simulink model "jav1pitch"  (R2025b)
settings: Solver=VariableStepAuto  StartTime=0.0  StopTime=41  RelTol=1e-3
undefined symbols (not defined in the file): Cd, delta_pitch_saturation, diameter, g, I_treghet, K_finne, Ki_altitude, Kp_altitude, L_aksial, m, rho, T, theta0, theta_dot, theta_ref_saturation, v_x0, v_z0, x0, z0, z_ref
libraries: slpidlib x2
settings Model: Creator=Tobias Stenberg  LastModifiedBy=kristiangjestad

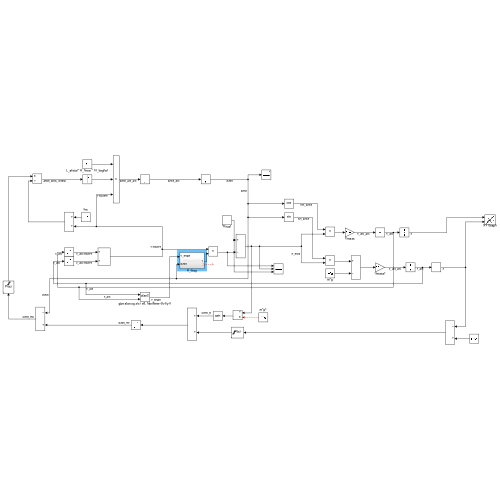
[thumbnail: Simulink's stored preview of the top-level diagram]
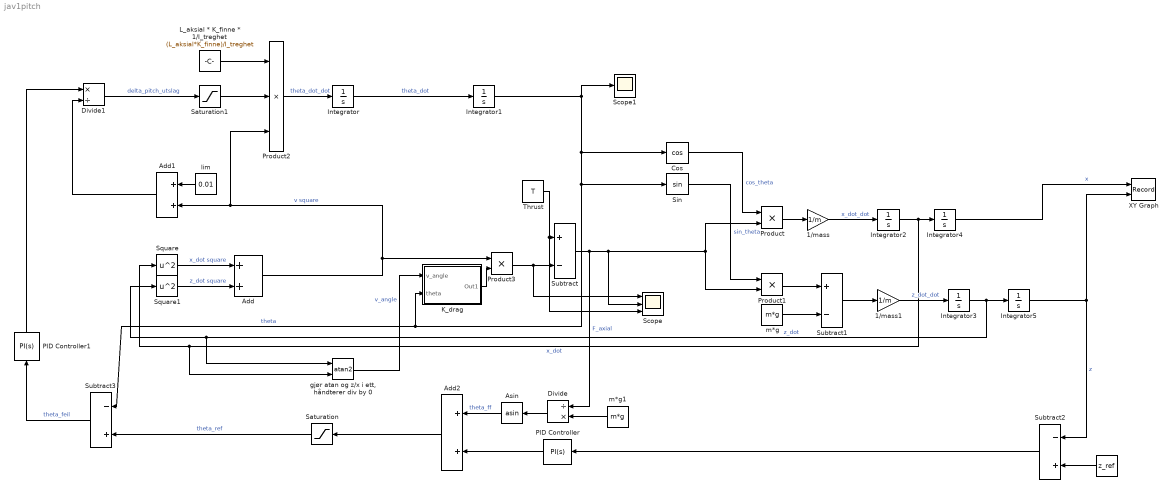
== system jav1pitch ==
  " " : Constant  Value=z_ref
  1/mass : Gain  Gain=1/m
  1/mass1 : Gain  Gain=1/m
  Add : Sum
  Add1 : Sum
  Add2 : Sum
  Asin : Trigonometry  Operator=asin
  Cos : Trigonometry  Operator=cos
  Divide : Product  Inputs=/*
  Divide1 : Product  Inputs=*/
  Integrator : Integrator  InitialCondition=theta_dot
  Integrator1 : Integrator  InitialCondition=theta0
  Integrator2 : Integrator  InitialCondition=v_x0
  Integrator3 : Integrator  InitialCondition=v_z0
  Integrator4 : Integrator  InitialCondition=x0
  Integrator5 : Integrator  InitialCondition=z0
  K_drag : Subsystem
  L_aksial * K_finne * 1/I_treghet : Constant  Value=(L_aksial*K_finne)/I_treghet
  PID Controller : slpidlib/PID Controller  Controller=PI  Form=Parallel  TimeDomain=Continuous-time  UseExternalTs=off  SampleTime=-1  IntegratorMethod=Forward Euler  FilterMethod=Forward Euler  ControllerParametersSource=internal  P=Kp_altitude  I=Ki_altitude  UseKiTs=off  D=0  UseExternalDerivativeSource=off  N=100  UseFilter=on  TunerSelectOption=Transfer Function Based (PID Tuner App)  InitialConditionSource=internal  InitialConditionForIntegrator=0  InitialConditionForFilter=0  DifferentiatorICPrevScaledInput=0  ExternalReset=none  TrackingMode=off  Kt=1  LimitOutput=on  SatLimitsSource=internal  UpperSaturationLimit=0.4  LowerSaturationLimit=-0.4  LinearizeAsGain=on  AntiWindupMode=clamping  Kb=1  LimitIntegrator=off  UpperIntegratorSaturationLimit=inf  LowerIntegratorSaturationLimit=-inf  POutMin=[]  POutMax=[]  IOutMin=[]  IOutMax=[]  DOutMin=[]  DOutMax=[]  NOutMin=[]  NOutMax=[]  SumOutMin=[]  SumOutMax=[]  SaturationOutMin=[]  SaturationOutMax=[]  PParamMin=[]  PParamMax=[]  IParamMin=[]  IParamMax=[]  DParamMin=[]  DParamMax=[]  NParamMin=[]  NParamMax=[]  KbParamMin=[]  KbParamMax=[]  KtParamMin=[]  KtParamMax=[]  KbOutMin=[]  KbOutMax=[]  KtOutMin=[]  KtOutMax=[]  IntegratorOutMin=[]  IntegratorOutMax=[]  FilterOutMin=[]  FilterOutMax=[]  SumI1OutMin=[]  SumI1OutMax=[]  SumI2OutMin=[]  SumI2OutMax=[]  SumI3OutMin=[]  SumI3OutMax=[]  SumI4OutMin=[]  SumI4OutMax=[]  SumDOutMin=[]  SumDOutMax=[]  DifferentiatorOutMin=[]  DifferentiatorOutMax=[]  FilterDiffOutCoefMin=[]  FilterDiffOutCoefMax=[]  ReciprocalOutMin=[]  ReciprocalOutMax=[]  SumDenOutMin=[]  SumDenOutMax=[]  SumNumOutMin=[]  SumNumOutMax=[]  DivideOutMin=[]  DivideOutMax=[]  UdiffTsProdOutMin=[]  UdiffTsProdOutMax=[]  NTsProdOutMin=[]  NTsProdOutMax=[]  UintegralTsProdOutMin=[]  UintegralTsProdOutMax=[]  UngainTsProdOutMin=[]  UngainTsProdOutMax=[]  ClampingZeroOutDataTypeStr=Inherit: Inherit via back propagation  ClampingZeroOutMin=[]  ClampingZeroOutMax=[]  FilterDenConstantOutDataTypeStr=Inherit: Inherit via back propagation  FilterDenConstantOutMin=[]  FilterDenConstantOutMax=[]  PCopyOutDataTypeStr=Inherit: Inherit via back propagation  PCopyOutMin=[]  PCopyOutMax=[]  NCopyOutDataTypeStr=Inherit: Inherit via back propagation  NCopyOutMin=[]  NCopyOutMax=[]  IntegratorContinuousStateAttributes=''  IntegratorStateMustResolveToSignalObject=off  IntegratorRTWStateStorageClass=Auto  FilterContinuousStateAttributes=''  FilterStateMustResolveToSignalObject=off  FilterRTWStateStorageClass=Auto  ParallelPVariant=InternalParameters  IdealPVariant=Disabled  IVariant=InternalParameters  DVariant=Disabled  IntegratorVariant=Continuous  SatVariant=Enabled  AWVariant=ContClampingParallel  PCopyVariant=Disabled  TRVariant=Disabled  FdbkBlocksVariant=Forward  IdealPFdbkVariant=Disabled  SatFdbkVariant=Disabled  DerivativeFilterVariant=Disabled  NVariant=Disabled  NCopyVariant=Disabled_SignalSpec  FilterICVariant=Disabled  IntegratorICVariant=InternalICs  ExternalResetVariant=Disabled  TRSumVariant=Passthrough  SumFdbkVariant=Disabled  SumVariant=Sum_PI  TsampFilterVariant=InternalTs  TsampNgainVariant=Passthrough  TsampIntegralVariant=Disabled_SignalSpec  ExternalSaturationOutDataTypeStr=Inherit: Same as second input  DerivativeSourceVariant=Disabled  PreIntVariant=InternalPreInt
  PID Controller1 : slpidlib/PID Controller  Controller=PI  Form=Parallel  TimeDomain=Continuous-time  UseExternalTs=off  SampleTime=-1  IntegratorMethod=Forward Euler  FilterMethod=Forward Euler  ControllerParametersSource=internal  P=Kp_altitude  I=Ki_altitude  UseKiTs=off  D=0  UseExternalDerivativeSource=off  N=100  UseFilter=on  TunerSelectOption=Transfer Function Based (PID Tuner App)  InitialConditionSource=internal  InitialConditionForIntegrator=0  InitialConditionForFilter=0  DifferentiatorICPrevScaledInput=0  ExternalReset=none  TrackingMode=off  Kt=1  LimitOutput=on  SatLimitsSource=internal  UpperSaturationLimit=0.4  LowerSaturationLimit=-0.4  LinearizeAsGain=on  AntiWindupMode=clamping  Kb=1  LimitIntegrator=off  UpperIntegratorSaturationLimit=inf  LowerIntegratorSaturationLimit=-inf  POutMin=[]  POutMax=[]  IOutMin=[]  IOutMax=[]  DOutMin=[]  DOutMax=[]  NOutMin=[]  NOutMax=[]  SumOutMin=[]  SumOutMax=[]  SaturationOutMin=[]  SaturationOutMax=[]  PParamMin=[]  PParamMax=[]  IParamMin=[]  IParamMax=[]  DParamMin=[]  DParamMax=[]  NParamMin=[]  NParamMax=[]  KbParamMin=[]  KbParamMax=[]  KtParamMin=[]  KtParamMax=[]  KbOutMin=[]  KbOutMax=[]  KtOutMin=[]  KtOutMax=[]  IntegratorOutMin=[]  IntegratorOutMax=[]  FilterOutMin=[]  FilterOutMax=[]  SumI1OutMin=[]  SumI1OutMax=[]  SumI2OutMin=[]  SumI2OutMax=[]  SumI3OutMin=[]  SumI3OutMax=[]  SumI4OutMin=[]  SumI4OutMax=[]  SumDOutMin=[]  SumDOutMax=[]  DifferentiatorOutMin=[]  DifferentiatorOutMax=[]  FilterDiffOutCoefMin=[]  FilterDiffOutCoefMax=[]  ReciprocalOutMin=[]  ReciprocalOutMax=[]  SumDenOutMin=[]  SumDenOutMax=[]  SumNumOutMin=[]  SumNumOutMax=[]  DivideOutMin=[]  DivideOutMax=[]  UdiffTsProdOutMin=[]  UdiffTsProdOutMax=[]  NTsProdOutMin=[]  NTsProdOutMax=[]  UintegralTsProdOutMin=[]  UintegralTsProdOutMax=[]  UngainTsProdOutMin=[]  UngainTsProdOutMax=[]  ClampingZeroOutDataTypeStr=Inherit: Inherit via back propagation  ClampingZeroOutMin=[]  ClampingZeroOutMax=[]  FilterDenConstantOutDataTypeStr=Inherit: Inherit via back propagation  FilterDenConstantOutMin=[]  FilterDenConstantOutMax=[]  PCopyOutDataTypeStr=Inherit: Inherit via back propagation  PCopyOutMin=[]  PCopyOutMax=[]  NCopyOutDataTypeStr=Inherit: Inherit via back propagation  NCopyOutMin=[]  NCopyOutMax=[]  IntegratorContinuousStateAttributes=''  IntegratorStateMustResolveToSignalObject=off  IntegratorRTWStateStorageClass=Auto  FilterContinuousStateAttributes=''  FilterStateMustResolveToSignalObject=off  FilterRTWStateStorageClass=Auto  ParallelPVariant=InternalParameters  IdealPVariant=Disabled  IVariant=InternalParameters  DVariant=Disabled  IntegratorVariant=Continuous  SatVariant=Enabled  AWVariant=ContClampingParallel  PCopyVariant=Disabled  TRVariant=Disabled  FdbkBlocksVariant=Forward  IdealPFdbkVariant=Disabled  SatFdbkVariant=Disabled  DerivativeFilterVariant=Disabled  NVariant=Disabled  NCopyVariant=Disabled_SignalSpec  FilterICVariant=Disabled  IntegratorICVariant=InternalICs  ExternalResetVariant=Disabled  TRSumVariant=Passthrough  SumFdbkVariant=Disabled  SumVariant=Sum_PI  TsampFilterVariant=InternalTs  TsampNgainVariant=Passthrough  TsampIntegralVariant=Disabled_SignalSpec  ExternalSaturationOutDataTypeStr=Inherit: Same as second input  DerivativeSourceVariant=Disabled  PreIntVariant=InternalPreInt
  Product : Product
  Product1 : Product
  Product2 : Product  Inputs=3
  Product3 : Product
  Saturation : Saturate  UpperLimit=theta_ref_saturation  LowerLimit=-theta_ref_saturation
  Saturation1 : Saturate  UpperLimit=delta_pitch_saturation  LowerLimit=-delta_pitch_saturation
  Scope : Scope  NumInputPorts=3
      settings: ActiveDisplayYMinimum=-272.68668201615378  ActiveDisplayYMaximum=1772.6866820161538
  Scope1 : Scope
      settings: ActiveDisplayYMinimum=-0.77176160217650369  ActiveDisplayYMaximum=0.51854075550484957
  Sin : Trigonometry
  Square : Math  Operator=square
  Square1 : Math  Operator=square
  Subtract : Sum  Inputs=+-
  Subtract1 : Sum  Inputs=+-
  Subtract2 : Sum  Inputs=-+
  Subtract3 : Sum  Inputs=-+
  Thrust : Constant  Value=T
  XY Graph : Record  NumPorts=2.0  FileSettingsInternal="{\"entries\":[{\"content\":{\"excelSettings\":{\"content\":{},\"type\":\"Streamout.ExcelSettings\"},\"parquetSettings\":{\"content\":{},\"type\":\"Streamout.ParquetSettings\"}},\"type\":\"Streamout.FileSettingStorage\",\"uuid\":\"\"}],\"packageUris\":[\"http:\\/\\/schema.mathworks.com\\/mf0\\/streamout_blocks\\/R2020a\"],\"version\":\"1.0\"}"  FrameSettings=[0, 0]  Layout=[1 1]  SignalsInternal="{\"entries\":[{\"content\":{\"signals\":[{\"content\":{\"blockPath\":[],\"dimensions\":[1],\"domain\":\"\",\"lineColor\":\"#a2142f\",\"port\":1,\"sid\":[\"\"],\"signalID\":1,\"signalName\":\"x\"},\"type\":\"RecordBlkView.Signal\",\"uuid\":\"\"},{\"content\":{\"blockPath\":[],\"dimensions\":[1],\"domain\":\"\",\"lineColor\":\"#139fff\",\"plots\":[ 1 ],\"port\":2,\"sid\":[\"\"],\"signalID\":2,\"signalName\":\"z\"},\"type\":\"RecordBlkView.Signal\",\"uuid\":\"\"}]},\"type\":\"RecordBlkView.InputSignals\",\"uuid\":\"\"}],\"packageUris\":[\"http:\\/\\/schema.mathworks.com\\/mf0\\/streamout_blocks\\/R2020a\"],\"version\":\"1.0\"}"  CompatibilityTag=XY
  "gjør atan og z/x i ett, håndterer div by 0" : Trigonometry  Operator=atan2
  lim : Constant  Value=0.01
  m*g : Constant  Value=m*g
  m*g1 : Constant  Value=m*g
  wires:
  Integrator/1 -> Integrator1/1  "theta_dot"
  Product2/1 -> Integrator/1  "theta_dot_dot"
  Integrator1/1 -> Sin/1, K_drag/2(theta), Subtract3/1, Cos/1, Scope1/1  "theta"
  Square/1 -> Add/1  "x_dot square"
  Square1/1 -> Add/2  "z_dot square"
  Add/1 -> Product2/3, Add1/2, Product3/1  "v square"
  Product3/1 -> Subtract/2, Scope/1
  Thrust/1 -> Scope/3, Subtract/1
  Subtract/1 -> Divide/1, Scope/2, Product1/2, Product/2  "F_axial"
  Cos/1 -> Product/1  "cos_theta"
  Sin/1 -> Product1/1  "sin_theta"
  Product1/1 -> Subtract1/1
  m*g/1 -> Subtract1/2
  Subtract1/1 -> 1/mass1/1
  1/mass1/1 -> Integrator3/1  "z_dot_dot"
  Product/1 -> 1/mass/1
  1/mass/1 -> Integrator2/1  "x_dot_dot"
  Integrator2/1 -> "gjør atan og z/x i ett, håndterer div by 0"/2, Square/1, Integrator4/1  "x_dot"
  Integrator3/1 -> "gjør atan og z/x i ett, håndterer div by 0"/1, Square1/1, Integrator5/1  "z_dot"
  Integrator4/1 -> XY Graph/1  "x"
  Integrator5/1 -> XY Graph/2, Subtract2/1  "z"
  L_aksial * K_finne * 1/I_treghet/1 -> Product2/1
  Divide1/1 -> Saturation1/1  "delta_pitch_utslag"
  m*g1/1 -> Divide/2
  Divide/1 -> Asin/1
  Asin/1 -> Add2/1  "theta_ff"
  lim/1 -> Add1/1
  Add1/1 -> Divide1/2
  Saturation/1 -> Subtract3/2  "theta_ref"
  Add2/1 -> Saturation/1
  " "/1 -> Subtract2/2
  PID Controller/1 -> Add2/2
  Subtract2/1 -> PID Controller/1
  Subtract3/1 -> PID Controller1/1  "theta_feil"
  Saturation1/1 -> Product2/2
  PID Controller1/1 -> Divide1/1
  "gjør atan og z/x i ett, håndterer div by 0"/1 -> K_drag/1(v_angle)  "v_angle"
  K_drag/1(Out1) -> Product3/2
  ? -> ?

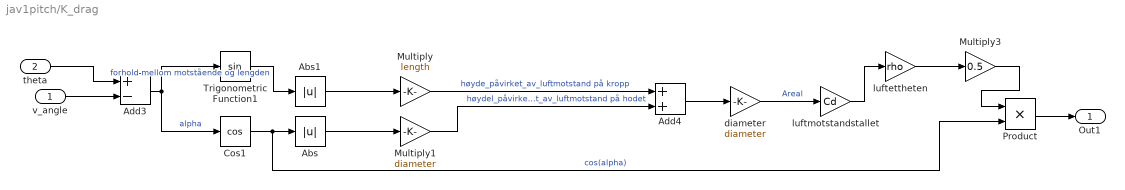
== system jav1pitch/K_drag ==
  v_angle : Inport
  theta : Inport  Port=2
  Abs : Abs  SaturateOnIntegerOverflow=off
  Abs1 : Abs  SaturateOnIntegerOverflow=off
  Add3 : Sum  Inputs=+-
  Add4 : Sum
  Cos1 : Trigonometry  Operator=cos
  Multiply : Gain  Gain=length
  Multiply1 : Gain  Gain=diameter
  Multiply3 : Gain  Gain=0.5
  Product : Product
  Trigonometric Function1 : Trigonometry
  diameter : Gain  Gain=diameter
  luftettheten : Gain  Gain=rho
  luftmotstandstallet : Gain  Gain=Cd
  Out1 : Outport
  wires:
  Multiply3/1 -> Product/1
  Multiply/1 -> Add4/1  "høyde_påvirket_av_luftmotstand på kropp"
  Add4/1 -> diameter/1
  theta/1 -> Add3/1
  Cos1/1 -> Product/2, Abs/1  "cos(alpha)"
  luftmotstandstallet/1 -> luftettheten/1
  v_angle/1 -> Add3/2
  Trigonometric Function1/1 -> Abs1/1  "forhold mellom motstående og lengden"
  diameter/1 -> luftmotstandstallet/1  "Areal"
  luftettheten/1 -> Multiply3/1
  Multiply1/1 -> Add4/2  "høydel_påvirket_av_luftmotstand på hodet"
  Add3/1 -> Cos1/1, Trigonometric Function1/1  "alpha"
  Abs1/1 -> Multiply/1
  Abs/1 -> Multiply1/1
  Product/1 -> Out1/1
